simulink model "ch7example27"  (Simulink 5.0)
settings: Solver=ode45  StartTime=0.0  StopTime=1000.0  MaxStep=1e-4  RelTol=1e-3
libraries: commutil2 x8, commdigbbndpm2 x4, commrandsrc2 x4, commseqgen2 x4, simulink x2, dspsigops x2, commchan2 x1
settings Model: LastModifiedBy=shaoyubin

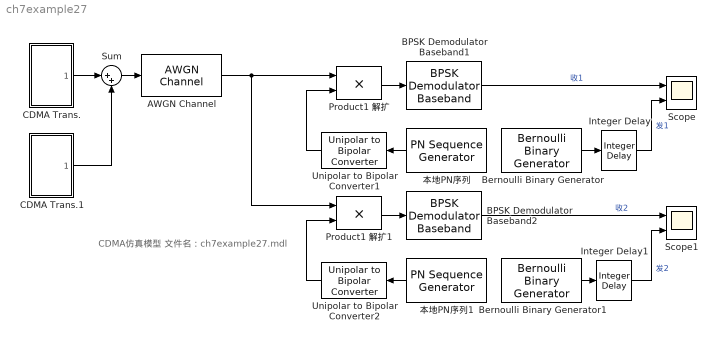
== system ch7example27 ==
  note: CDMA仿真模型
      | 文件名：ch7example27.mdl
  AWGN Channel : commchan2/AWGN Channel  seed=67  noiseMode=Variance from mask  EsNodB=10  SNRdB=10  Ps=1  Tsym=1  variance=5
  BPSK Demodulator Baseband1 : commdigbbndpm2/BPSK Demodulator Baseband  Ph=0  numSamp=20
  BPSK Demodulator Baseband2 : commdigbbndpm2/BPSK Demodulator Baseband  Ph=0  numSamp=20
  Bernoulli Binary Generator : commrandsrc2/Bernoulli Binary Generator  P=0.5  seed=61  Ts=1/100  frameBased=off  sampPerFrame=1  orient=off
  Bernoulli Binary Generator1 : commrandsrc2/Bernoulli Binary Generator  P=0.5  seed=77  Ts=1/100  frameBased=off  sampPerFrame=1  orient=off
  CDMA Trans. : Subsystem
  CDMA Trans.1 : Subsystem
  Integer Delay : dspsigops/Integer Delay  delay=2  ic=0  reset_popup=None
  Integer Delay1 : dspsigops/Integer Delay  delay=2  ic=0  reset_popup=None
  Product1 解扩 : Product  SaturateOnIntegerOverflow=on
  Product1 解扩1 : Product  SaturateOnIntegerOverflow=on
  Scope : Scope  NumInputPorts=2
      settings: TimeRange=0.4  YMin=-2~-2  YMax=2~2
  Scope1 : Scope  NumInputPorts=2
      settings: TimeRange=0.4  YMin=-2~-2  YMax=2~2
  Sum : Sum  Inputs=|++  SaturateOnIntegerOverflow=on
  Unipolar to Bipolar Converter1 : commutil2/Unipolar to Bipolar Converter  Orientation=left  M=2  polarity=Positive
  Unipolar to Bipolar Converter2 : commutil2/Unipolar to Bipolar Converter  Orientation=left  M=2  polarity=Positive
  本地PN序列 : commseqgen2/PN Sequence Generator  Orientation=left  poly=[1 0 0 0 0 1 1]  ini_sta=[0 0 0 0 0 1]  shift=0  Ts=1/2000  frameBased=off  sampPerFrame=1  reset=off
  本地PN序列1 : commseqgen2/PN Sequence Generator  Orientation=left  poly=[1 0 0 0 0 1 1]  ini_sta=[0 0 0 0 1 1]  shift=0  Ts=1/2000  frameBased=off  sampPerFrame=1  reset=off
  wires:
  本地PN序列/1 -> Unipolar to Bipolar Converter1/1
  Product1 解扩/1 -> BPSK Demodulator Baseband1/1
  CDMA Trans./1(CDMA) -> Sum/1
  Sum/1 -> AWGN Channel/1
  CDMA Trans.1/1(CDMA) -> Sum/2
  Unipolar to Bipolar Converter1/1 -> Product1 解扩/2
  AWGN Channel/1 -> Product1 解扩/1, Product1 解扩1/1
  Bernoulli Binary Generator/1 -> Integer Delay/1
  BPSK Demodulator Baseband1/1 -> Scope/1  "收1"
  Integer Delay/1 -> Scope/2  "发1"
  本地PN序列1/1 -> Unipolar to Bipolar Converter2/1
  Product1 解扩1/1 -> BPSK Demodulator Baseband2/1
  Unipolar to Bipolar Converter2/1 -> Product1 解扩1/2
  Bernoulli Binary Generator1/1 -> Integer Delay1/1
  BPSK Demodulator Baseband2/1 -> Scope1/1  "收2"
  Integer Delay1/1 -> Scope1/2  "发2"

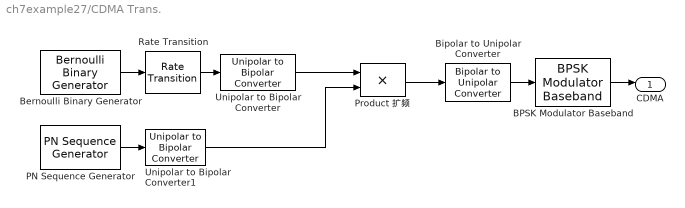
== system ch7example27/CDMA Trans. ==
  BPSK Modulator Baseband : commdigbbndpm2/BPSK Modulator Baseband  Ph=0  numSamp=1
  Bernoulli Binary Generator : commrandsrc2/Bernoulli Binary Generator  P=0.5  seed=61  Ts=1/100  frameBased=off  sampPerFrame=1  orient=off
  Bipolar to Unipolar Converter : commutil2/Bipolar to Unipolar Converter  M=2  polarity=Positive
  PN Sequence Generator : commseqgen2/PN Sequence Generator  poly=[1 0 0 0 0 1 1]  ini_sta=[0 0 0 0 0 1]  shift=0  Ts=1/2000  frameBased=off  sampPerFrame=1  reset=off
  Product 扩频 : Product  SaturateOnIntegerOverflow=on
  Rate Transition : simulink/Signal Attributes/Rate Transition  DataIntegrity=on  DeterministicTransfer=on  TransitionType=Slow to fast  InitCond=0
  Unipolar to Bipolar Converter : commutil2/Unipolar to Bipolar Converter  M=2  polarity=Positive
  Unipolar to Bipolar Converter1 : commutil2/Unipolar to Bipolar Converter  M=2  polarity=Positive
  CDMA : Outport
  wires:
  Bernoulli Binary Generator/1 -> Rate Transition/1
  PN Sequence Generator/1 -> Unipolar to Bipolar Converter1/1
  Product 扩频/1 -> Bipolar to Unipolar Converter/1
  Unipolar to Bipolar Converter/1 -> Product 扩频/1
  Bipolar to Unipolar Converter/1 -> BPSK Modulator Baseband/1
  Unipolar to Bipolar Converter1/1 -> Product 扩频/2
  Rate Transition/1 -> Unipolar to Bipolar Converter/1
  BPSK Modulator Baseband/1 -> CDMA/1

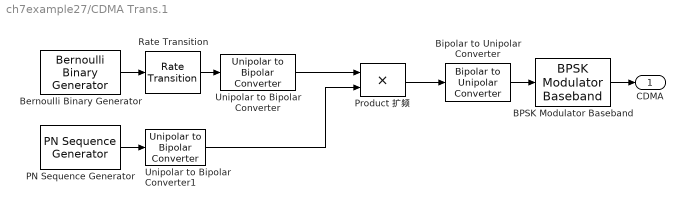
== system ch7example27/CDMA Trans.1 ==
  BPSK Modulator Baseband : commdigbbndpm2/BPSK Modulator Baseband  Ph=0  numSamp=1
  Bernoulli Binary Generator : commrandsrc2/Bernoulli Binary Generator  P=0.5  seed=77  Ts=1/100  frameBased=off  sampPerFrame=1  orient=off
  Bipolar to Unipolar Converter : commutil2/Bipolar to Unipolar Converter  M=2  polarity=Positive
  PN Sequence Generator : commseqgen2/PN Sequence Generator  poly=[1 0 0 0 0 1 1]  ini_sta=[0 0 0 0 1 1]  shift=0  Ts=1/2000  frameBased=off  sampPerFrame=1  reset=off
  Product 扩频 : Product  SaturateOnIntegerOverflow=on
  Rate Transition : simulink/Signal Attributes/Rate Transition  DataIntegrity=on  DeterministicTransfer=on  TransitionType=Slow to fast  InitCond=0
  Unipolar to Bipolar Converter : commutil2/Unipolar to Bipolar Converter  M=2  polarity=Positive
  Unipolar to Bipolar Converter1 : commutil2/Unipolar to Bipolar Converter  M=2  polarity=Positive
  CDMA : Outport
  wires:
  BPSK Modulator Baseband/1 -> CDMA/1
  Rate Transition/1 -> Unipolar to Bipolar Converter/1
  Unipolar to Bipolar Converter1/1 -> Product 扩频/2
  Bipolar to Unipolar Converter/1 -> BPSK Modulator Baseband/1
  Unipolar to Bipolar Converter/1 -> Product 扩频/1
  Product 扩频/1 -> Bipolar to Unipolar Converter/1
  PN Sequence Generator/1 -> Unipolar to Bipolar Converter1/1
  Bernoulli Binary Generator/1 -> Rate Transition/1
